simulink model "some_model"  (R2023b)
settings: Solver=VariableStepAuto  StartTime=0.0  StopTime=10.0  RelTol=1e-3
settings Model: Creator=henryyost  LastModifiedBy=henryyost

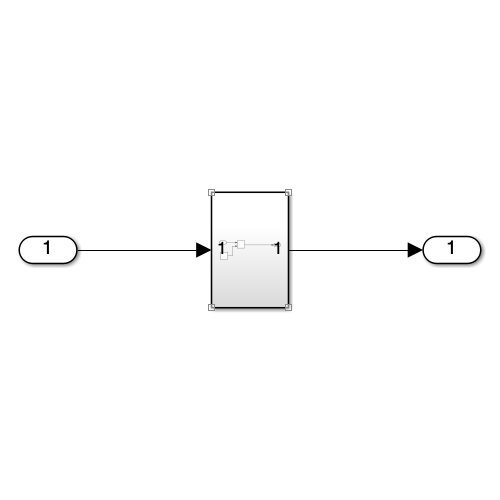
[thumbnail: Simulink's stored preview of the top-level diagram]
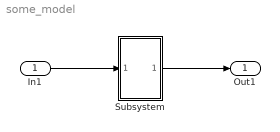
== system some_model ==
  In1 : Inport
  Subsystem : Subsystem
  Out1 : Outport
  wires:
  In1/1 -> Subsystem/1(In1)
  Subsystem/1(Out1) -> Out1/1

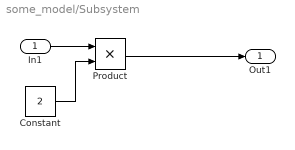
== system some_model/Subsystem ==
  In1 : Inport
  Constant : Constant  Value=2
  Product : Product
  Out1 : Outport
  wires:
  Product/1 -> Out1/1
  In1/1 -> Product/1
  Constant/1 -> Product/2
